simulink model "sampleModel1854"  (R2023a)
settings: Solver=VariableStepAuto  StartTime=0.0  StopTime=10.0  RelTol=1e-3
libraries: hdlsllib x7, simulink x2
settings Model: Creator=user1  LastModifiedBy=user1

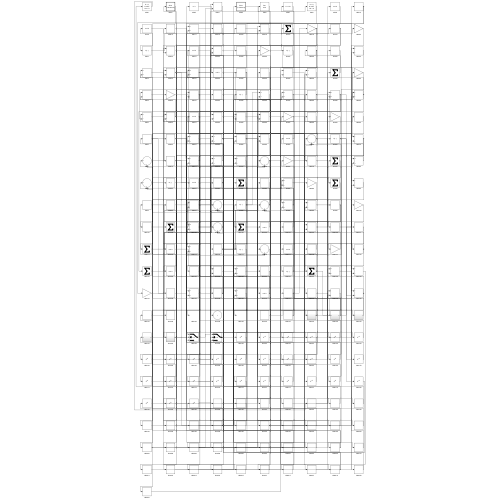
[thumbnail: Simulink's stored preview of the top-level diagram]
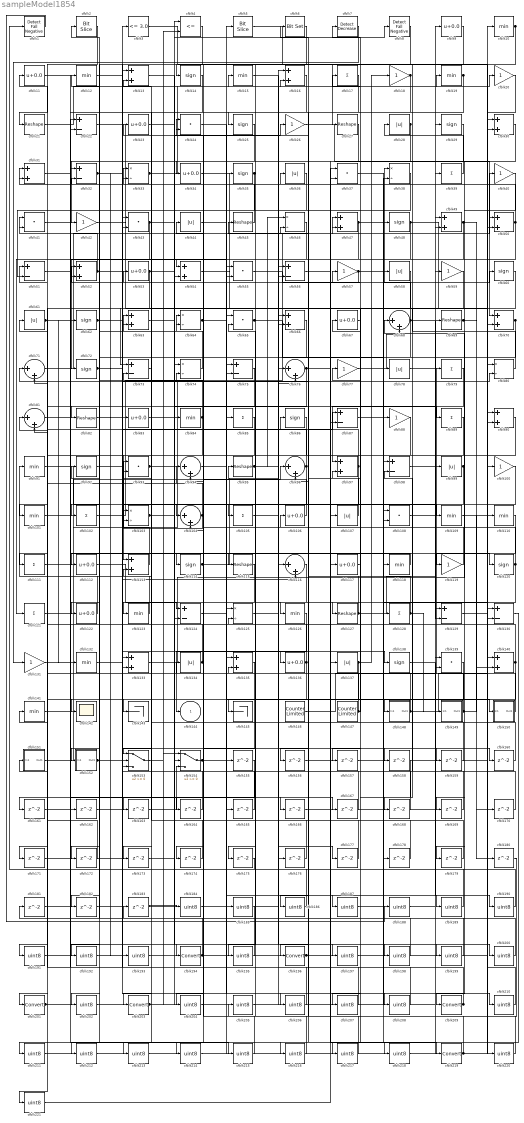
== system sampleModel1854 ==
  cfblk1 : hdlsllib/Logic and Bit Operations/Detect Fall Negative  vinit=0  OutDataTypeStr=boolean
  cfblk{10,12,15,19,84,91,101,109..110,118,123,126,132,141} (14 alike) : MinMax
  cfblk{18,20,26,40,42,57,59,77,88,100,119,131} (12 alike) : Gain
  cfblk{17,39,79,85,89,102,105,111,121,128} (10 alike) : Sum  Inputs=+
  cfblk{33,38,46,64,74,80,103,125} (8 alike) : Product  Inputs=*/  RndMeth=Zero  SaturateOnIntegerOverflow=on
  cfblk{68,71,76,81,94,96,104,116} (8 alike) : Sum  Inputs=|++
  cfblk{9,11,23,34,53,67,83,106,112,117,122,136} (12 alike) : Bias  Bias=0.0  SaturateOnIntegerOverflow=off
  cfblk{28,36,44,58,61,78,99,107,134,137} (10 alike) : Abs  SaturateOnIntegerOverflow=off
  cfblk{24,37,41,43,55,65,93,108,139} (9 alike) : DotProduct  OutDataTypeStr=Inherit: Inherit via internal rule
  cfblk{13,16,30..31,47,49..50,52,54,63,66,70,90,97,113,133,135,140} (18 alike) : Sum
  cfblk{14,25,29,35,48,60,62,72,86,92,114,120,138} (13 alike) : Signum
  cfblk{21,27,45,69,82,95,115,127} (8 alike) : Reshape
  cfblk{22,32,51,56,73,75,87,98,124,129..130} (11 alike) : Sum  Inputs=+-
  cfblk142 : Scope
  cfblk143 : Terminator
  cfblk145 : Terminator
  cfblk146 : hdlsllib/Sources/Counter Limited  uplimit=7  tsamp=-1
  cfblk147 : hdlsllib/Sources/Counter Limited  uplimit=7  tsamp=-1
  cfblk148 : Subsystem
      settings: LibrarySourceBlock=|
      | hdlsllib/Ports &
      | Subsystems/Subsystem
  cfblk149 : Subsystem
      settings: LibrarySourceBlock=|
      | hdlsllib/Ports &
      | Subsystems/Subsystem
  cfblk150 : Subsystem
      settings: LibrarySourceBlock=|
      | hdlsllib/Ports &
      | Subsystems/Subsystem
  cfblk151 : Subsystem
      settings: LibrarySourceBlock=|
      | hdlsllib/Ports &
      | Subsystems/Subsystem
  cfblk152 : Subsystem
      settings: LibrarySourceBlock=|
      | hdlsllib/Ports &
      | Subsystems/Subsystem
  cfblk153 : Switch  SaturateOnIntegerOverflow=off  InputSameDT=off
  cfblk154 : Switch  SaturateOnIntegerOverflow=off  InputSameDT=off
  cfblk{155..183} (29 alike) : Delay  SampleTime=1
  cfblk{184..193,195,197..200,202,204..208,210..218,220..221} (32 alike) : DataTypeConversion  OutDataTypeStr=uint8  SaturateOnIntegerOverflow=off  RndMeth=Floor
  cfblk{194,196,201,203,209,219} (6 alike) : DataTypeConversion  SaturateOnIntegerOverflow=off  RndMeth=Floor
  cfblk2 : hdlsllib/Logic and Bit Operations/Bit Slice  lidx=7  ridx=0
  cfblk3 : hdlsllib/Logic and Bit Operations/Compare To Constant  relop=<=  const=3.0  OutDataTypeStr=boolean
  cfblk4 : RelationalOperator  Operator=<=  OutDataTypeStr=boolean  InputSameDT=off
  cfblk5 : hdlsllib/Logic and Bit Operations/Bit Slice  lidx=7  ridx=0
  cfblk6 : simulink/Logic and Bit Operations/Bit Set  iBit=0
      settings: LibrarySourceBlock=|
      | hdlsllib/Logic and Bit
      | Operations/Bit Set
  cfblk7 : simulink/Logic and Bit Operations/Detect Decrease  vinit=0.0  OutDataTypeStr=boolean
      settings: LibrarySourceBlock=|
      | hdlsllib/Logic and Bit
      | Operations/Detect
      | Decrease
  cfblk8 : hdlsllib/Logic and Bit Operations/Detect Fall Negative  vinit=0  OutDataTypeStr=boolean
  cfblk144 : Outport  VectorParamsAs1DForOutWhenUnconnected=off
  wires:
  cfblk119/1 -> cfblk63/1
  cfblk79/1 -> cfblk97/1
  cfblk80/1 -> cfblk73/1
  cfblk21/1 -> cfblk15/1
  cfblk133/1 -> cfblk68/1
  cfblk68/1 -> cfblk38/1, cfblk130/2, cfblk182/1
  cfblk111/1 -> cfblk96/1
  cfblk146/1 -> cfblk79/1
  cfblk117/1 -> cfblk57/1
  cfblk122/1 -> cfblk91/1
  cfblk34/1 -> cfblk117/1
  cfblk26/1 -> cfblk70/1
  cfblk137/1 -> cfblk18/1, cfblk161/1
  cfblk141/1 -> cfblk194/1
  cfblk99/1 -> cfblk126/1, cfblk157/1
  cfblk40/1 -> cfblk119/1
  cfblk140/1 -> cfblk33/1, cfblk171/1
  cfblk150/1(Out1) -> cfblk77/1
  cfblk43/1 -> cfblk121/1, cfblk19/1
  cfblk33/1 -> cfblk20/1, cfblk136/1
  cfblk25/1 -> cfblk42/1
  cfblk18/1 -> cfblk202/1, cfblk216/1
  cfblk20/1 -> cfblk70/2
  cfblk88/1 -> cfblk201/1
  cfblk126/1 -> cfblk144/1
  cfblk47/1 -> cfblk118/1, cfblk143/1
  cfblk7/1 -> cfblk131/1
  cfblk112/1 -> cfblk124/1
  cfblk19/1 -> cfblk123/1, cfblk22/2
  cfblk10/1 -> cfblk82/1, cfblk175/1
  cfblk51/1 -> cfblk32/1
  cfblk136/1 -> cfblk51/1, cfblk53/1, cfblk174/1
  cfblk96/1 -> cfblk61/1, cfblk64/1, cfblk103/1
  cfblk153/1 -> cfblk154/1
  cfblk14/1 -> cfblk102/1
  cfblk71/1 -> cfblk40/1
  cfblk90/1 -> cfblk127/1
  cfblk37/1 -> cfblk219/1
  cfblk72/1 -> cfblk120/1, cfblk193/1
  cfblk76/1 -> cfblk153/1, cfblk218/1
  cfblk30/1 -> cfblk209/1
  cfblk48/1 -> cfblk72/1, cfblk140/1
  cfblk102/1 -> cfblk35/1
  cfblk151/1(Out1) -> cfblk86/1
  cfblk148/1(Out1) -> cfblk31/1, cfblk90/2
  cfblk82/1 -> cfblk63/2
  cfblk128/1 -> cfblk71/1, cfblk149/1(In1)
  cfblk93/1 -> cfblk48/1, cfblk26/1
  cfblk49/1 -> cfblk152/1(In1), cfblk180/1, cfblk213/1
  cfblk78/1 -> cfblk39/1
  cfblk31/1 -> cfblk62/1
  cfblk22/1 -> cfblk137/1
  cfblk5/1 -> cfblk27/1
  cfblk98/1 -> cfblk69/1
  cfblk77/1 -> cfblk68/2
  cfblk66/1 -> cfblk203/1
  cfblk123/1 -> cfblk31/2
  cfblk108/1 -> cfblk29/1
  cfblk152/1(Out1) -> cfblk16/2, cfblk164/1
  cfblk121/1 -> cfblk5/1
  cfblk54/1 -> cfblk108/2
  cfblk61/1 -> cfblk114/1, cfblk132/1
  cfblk120/1 -> cfblk6/1, cfblk153/2
  cfblk70/1 -> cfblk115/1, cfblk172/1
  cfblk89/1 -> cfblk111/1
  cfblk131/1 -> cfblk95/1
  cfblk46/1 -> cfblk104/1
  cfblk86/1 -> cfblk113/1
  cfblk42/1 -> cfblk78/1
  cfblk106/1 -> cfblk24/1
  cfblk17/1 -> cfblk25/1
  cfblk114/1 -> cfblk76/1, cfblk47/1, cfblk47/2
  cfblk107/1 -> cfblk45/1
  cfblk147/1 -> cfblk97/2, cfblk104/2
  cfblk127/1 -> cfblk99/1, cfblk23/1
  cfblk124/1 -> cfblk50/1
  cfblk118/1 -> cfblk112/1
  cfblk109/1 -> cfblk10/1
  cfblk69/1 -> cfblk140/2, cfblk169/1, cfblk170/1
  cfblk65/1 -> cfblk128/1, cfblk167/1
  cfblk84/1 -> cfblk2/1, cfblk122/1
  cfblk74/1 -> cfblk12/1
  cfblk55/1 -> cfblk60/1
  cfblk45/1 -> cfblk11/1
  cfblk64/1 -> cfblk150/1(In1), cfblk208/1
  cfblk67/1 -> cfblk17/1
  cfblk35/1 -> cfblk54/1, cfblk145/1
  cfblk36/1 -> cfblk142/1
  cfblk104/1 -> cfblk81/1, cfblk103/2
  cfblk6/1 -> cfblk34/1
  cfblk58/1 -> cfblk81/2
  cfblk149/1(Out1) -> cfblk7/1, cfblk67/1, cfblk110/1
  cfblk57/1 -> cfblk129/2, cfblk52/2
  cfblk134/1 -> cfblk74/2, cfblk52/1
  cfblk132/1 -> cfblk87/1
  cfblk113/1 -> cfblk93/1
  cfblk2/1 -> cfblk21/1
  cfblk39/1 -> cfblk28/1
  cfblk56/1 -> cfblk148/1(In1)
  cfblk11/1 -> cfblk55/2
  cfblk8/1 -> cfblk14/1
  cfblk13/1 -> cfblk89/1
  cfblk91/1 -> cfblk116/1
  cfblk16/1 -> cfblk56/2
  cfblk28/1 -> cfblk87/2, cfblk192/1
  cfblk92/1 -> cfblk80/2
  cfblk154/1 -> cfblk64/2, cfblk155/1
  cfblk3/1 -> cfblk90/1
  cfblk100/1 -> cfblk196/1
  cfblk95/1 -> cfblk109/1, cfblk46/1
  cfblk103/1 -> cfblk84/1, cfblk105/1
  cfblk52/1 -> cfblk130/1, cfblk41/1
  cfblk32/1 -> cfblk3/1, cfblk83/1, cfblk159/1
  cfblk97/1 -> cfblk36/1, cfblk46/2, cfblk153/3
  cfblk73/1 -> cfblk13/2
  cfblk38/1 -> cfblk51/2
  cfblk53/1 -> cfblk8/1, cfblk101/1
  cfblk4/1 -> cfblk133/2
  cfblk116/1 -> cfblk124/2
  cfblk50/1 -> cfblk32/2, cfblk195/1
  cfblk62/1 -> cfblk116/2, cfblk138/1
  cfblk29/1 -> cfblk156/1
  cfblk156/1 -> cfblk80/1
  cfblk157/1 -> cfblk38/2
  cfblk23/1 -> cfblk158/1
  cfblk159/1 -> cfblk93/2
  cfblk83/1 -> cfblk160/1
  cfblk160/1 -> cfblk129/1
  cfblk161/1 -> cfblk74/1
  cfblk81/1 -> cfblk162/1
  cfblk60/1 -> cfblk163/1
  cfblk163/1 -> cfblk154/3
  cfblk164/1 -> cfblk13/1
  cfblk165/1 -> cfblk73/2
  cfblk41/1 -> cfblk166/1
  cfblk166/1 -> cfblk49/1
  cfblk167/1 -> cfblk56/1
  cfblk9/1 -> cfblk168/1
  cfblk168/1 -> cfblk65/2
  cfblk169/1 -> cfblk133/1
  cfblk170/1 -> cfblk98/2
  cfblk171/1 -> cfblk4/1
  cfblk172/1 -> cfblk71/2
  cfblk115/1 -> cfblk173/1
  cfblk174/1 -> cfblk33/2
  cfblk175/1 -> cfblk1/1
  cfblk15/1 -> cfblk176/1
  cfblk176/1 -> cfblk113/2
  cfblk105/1 -> cfblk177/1
  cfblk177/1 -> cfblk16/1
  cfblk87/1 -> cfblk178/1
  cfblk178/1 -> cfblk154/2
  cfblk110/1 -> cfblk179/1
  cfblk179/1 -> cfblk96/2
  cfblk181/1 -> cfblk43/2
  cfblk182/1 -> cfblk76/2
  cfblk183/1 -> cfblk184/1
  cfblk24/1 -> cfblk185/1
  cfblk185/1 -> cfblk183/1
  cfblk139/1 -> cfblk186/1
  cfblk186/1 -> cfblk151/1(In1)
  cfblk184/1 -> cfblk187/1
  cfblk187/1 -> cfblk139/1
  cfblk1/1 -> cfblk188/1
  cfblk188/1 -> cfblk139/2
  cfblk44/1 -> cfblk189/1
  cfblk189/1 -> cfblk65/1
  cfblk138/1 -> cfblk190/1
  cfblk190/1 -> cfblk44/1
  cfblk75/1 -> cfblk191/1
  cfblk191/1 -> cfblk50/2
  cfblk192/1 -> cfblk75/1
  cfblk193/1 -> cfblk75/2
  cfblk194/1 -> cfblk165/1, cfblk41/2
  cfblk195/1 -> cfblk141/1
  cfblk196/1 -> cfblk98/1, cfblk9/1
  cfblk63/1 -> cfblk197/1
  cfblk197/1 -> cfblk100/1
  cfblk125/1 -> cfblk198/1
  cfblk198/1 -> cfblk92/1
  cfblk173/1 -> cfblk199/1
  cfblk199/1 -> cfblk125/1
  cfblk12/1 -> cfblk200/1
  cfblk200/1 -> cfblk125/2
  cfblk201/1 -> cfblk49/2, cfblk58/1
  cfblk202/1 -> cfblk88/1
  cfblk203/1 -> cfblk54/2, cfblk4/2, cfblk108/1
  cfblk27/1 -> cfblk204/1
  cfblk204/1 -> cfblk66/1
  cfblk180/1 -> cfblk205/1
  cfblk205/1 -> cfblk66/2
  cfblk94/1 -> cfblk206/1
  cfblk206/1 -> cfblk43/1
  cfblk158/1 -> cfblk207/1
  cfblk207/1 -> cfblk94/1
  cfblk208/1 -> cfblk94/2
  cfblk209/1 -> cfblk181/1, cfblk22/1
  cfblk162/1 -> cfblk210/1
  cfblk210/1 -> cfblk30/1
  cfblk130/1 -> cfblk211/1
  cfblk211/1 -> cfblk30/2
  cfblk85/1 -> cfblk212/1
  cfblk212/1 -> cfblk107/1
  cfblk213/1 -> cfblk85/1
  cfblk135/1 -> cfblk214/1
  cfblk214/1 -> cfblk55/1
  cfblk101/1 -> cfblk215/1
  cfblk215/1 -> cfblk135/1
  cfblk216/1 -> cfblk135/2
  cfblk59/1 -> cfblk217/1
  cfblk217/1 -> cfblk106/1
  cfblk218/1 -> cfblk59/1
  cfblk219/1 -> cfblk24/2, cfblk134/1
  cfblk129/1 -> cfblk220/1
  cfblk220/1 -> cfblk37/1
  cfblk155/1 -> cfblk221/1
  cfblk221/1 -> cfblk37/2

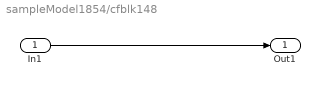
== system sampleModel1854/cfblk148 ==
  In1 : Inport
  Out1 : Outport
  wires:
  In1/1 -> Out1/1

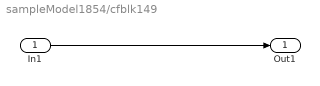
== system sampleModel1854/cfblk149 ==
  In1 : Inport
  Out1 : Outport
  wires:
  In1/1 -> Out1/1

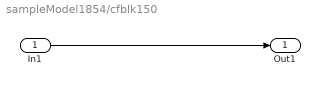
== system sampleModel1854/cfblk150 ==
  In1 : Inport
  Out1 : Outport
  wires:
  In1/1 -> Out1/1

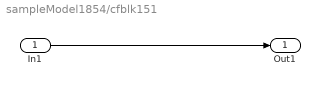
== system sampleModel1854/cfblk151 ==
  In1 : Inport
  Out1 : Outport
  wires:
  In1/1 -> Out1/1

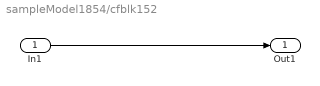
== system sampleModel1854/cfblk152 ==
  In1 : Inport
  Out1 : Outport
  wires:
  In1/1 -> Out1/1
